simulink model "safecomp_demo_pre"  (R2024a)
settings: Solver=ode4  StartTime=0  StopTime=15  FixedStep=0.1  RelTol=1e-3
undefined symbols (not defined in the file): Defined, Ego, Lane, User
libraries: roadrunnerscenario x3
settings Model: Creator=matsulab  LastModifiedBy=matsulab

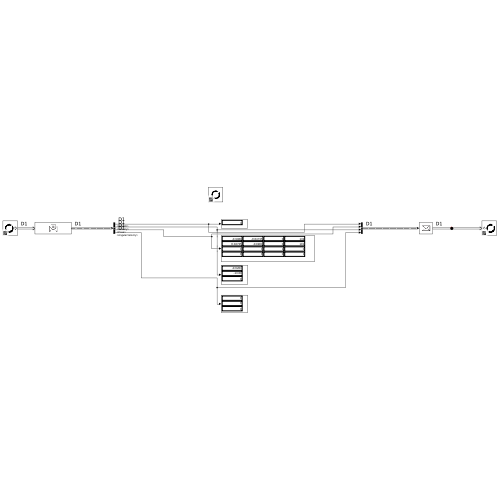
[thumbnail: Simulink's stored preview of the top-level diagram]
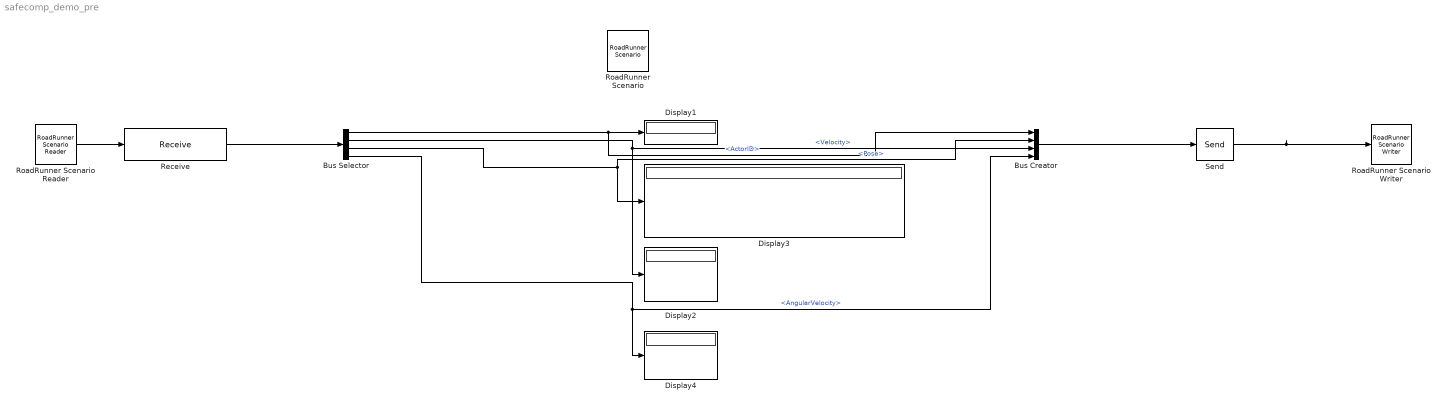
== system safecomp_demo_pre ==
  Bus Creator : BusCreator  Inputs=4  OutDataTypeStr=Bus: BusActorRuntime  NonVirtualBus=on
  Bus Selector : BusSelector  OutputSignals=ActorID,Velocity,Pose,AngularVelocity
  Display{1..4} (4 alike) : Display
  Receive : Receive  InputPortMessageModes=m  UseInternalQueue=off  QueueOverwriting=on  QueueLength=1  QueueType=LIFO
  RoadRunner Scenario : roadrunnerscenario/RoadRunner Scenario  UserDefinedActions={}  UserDefinedEvents={}
  RoadRunner Scenario Reader : roadrunnerscenario/RoadRunner Scenario Reader  TopicCategory=Actor  ActorCategory=All Types  ActionType=Speed Change  EventType=User-Defined  TopicType=Actor Pose  VehicleType=Vehicle Specifications  UserDefinedAction=Action1  UserDefinedEvent=Event1  Filter=Self  SensorTopic=Target Poses  LaneBoundaryOutputTopic=Ego-Lane  SensorID=1  SampleTime=0
  RoadRunner Scenario Writer : roadrunnerscenario/RoadRunner Scenario Writer  TopicCategory=Actor  ActorCategory=All Types  EventType=Action Complete  UserDefinedEvent=Event1  VehicleType=Vehicle Pose  TopicType=Actor Pose
  Send : Send  OutputPortMessageModes=m
  wires:
  RoadRunner Scenario Reader/1 -> Receive/1
  Receive/1 -> Bus Selector/1
  Bus Selector/1 -> Bus Creator/1, Display1/1  "<ActorID>"
  Send/1 -> RoadRunner Scenario Writer/1
  Bus Selector/2 -> Display2/1, Bus Creator/3  "<Velocity>"
  Bus Selector/4 -> Bus Creator/4, Display4/1  "<AngularVelocity>"
  Bus Selector/3 -> Display3/1, Bus Creator/2  "<Pose>"
  Bus Creator/1 -> Send/1
